simulink model "SecRwLtStHdrstFwdBkwdCtrl"  (R2018b)
settings: Solver=FixedStepDiscrete  StartTime=0.0  StopTime=10.0  FixedStep=0.01  RelTol=1e-3
undefined symbols (not defined in the file or in its folder): KeSMSuMdMotFinshdTm_Val, KeSMSuMdRetryTm1_Val, KeSMSuModeReqDurgTm_Val, KeSMSwSecRwLtStHdrstFwdBkwdEnTrigBitMask_Val
libraries: StCtrlLib x1
settings Model: Creator=sn2xws  LastModifiedBy=sn2xws
settings DataIOCC: SaveFormat=StructureWithTime
settings OptimizationCC: DefaultParameterBehavior=Inlined  EnhancedBackFolding=on  PassReuseOutputArgsAs=Individual arguments  ZeroExternalMemoryAtStartup=off  ZeroInternalMemoryAtStartup=off  OptimizeBlockOrder=speed  DifferentSizesBufferReuse=on  OptimizationCustomize=off
settings DebuggingCC: ParameterTunabilityLossMsg=error
settings ModelReferenceCC: ModelReferenceNumInstancesAllowed=Single
settings SFSimCC: MATLABDynamicMemAlloc=off
settings RTWCC: SystemTargetFile=autosar.tlc  GenCodeOnly=on  TemplateMakefile=ert_default_tmf  Description=AUTOSAR  GenerateReport=on  IncludeHyperlinkInReport=on  LaunchReport=on  GenerateTraceInfo=on  GenerateTraceReport=on  GenerateTraceReportSl=on  GenerateTraceReportSf=on  GenerateTraceReportEml=on
settings CodeAppCC: ForceParamTrailComments=on  IgnoreCustomStorageClasses=off  OperatorAnnotations=on  SimulinkDataObjDesc=on  SFDataObjDesc=on  InsertBlockDesc=on
settings STFCustomTargetCC: TargetLangStandard=C99 (ISO)  MultiwordLength=256  ParMdlRefBuildCompliant=on  CompOptLevelCompliant=on  IncludeMdlTerminateFcn=off  CombineOutputUpdateFcns=on  SuppressErrorStatus=on  ERTCustomFileBanners=on  SupportNonFinite=off  SupportComplex=off  SupportContinuousTime=off  SupportNonInlinedSFcns=off  RemoveResetFunc=on  MATLABClassNameForMDSCustomization=Simulink.SoftwareTarget.ERTCustomization  AutosarCompliant=on  UseToolchainInfoCompliant=on  LookupTableObjectStructAxisOrder=2,1,3,4,...  LUTObjectStructOrderEvenSpacing=Size,Table,Breakpoints  SystemTargetFile=autosar.tlc
settings ERTTargetCC: TargetLangStandard=C99 (ISO)  ConcurrentExecutionCompliant=off  IncludeMdlTerminateFcn=off  SuppressErrorStatus=on  SupportNonFinite=off  SupportComplex=off  ModelStepFunctionPrototypeControlCompliant=off  CPPClassGenCompliant=off  AutosarCompliant=on  LookupTableObjectStructAxisOrder=2,1,3,4,...  LUTObjectStructOrderEvenSpacing=Size,Table,Breakpoints  InlinedParameterPlacement=NonHierarchical  ERTCustomFileTemplate=example_file_process.tlc  ERTFilePackagingFormat=Compact

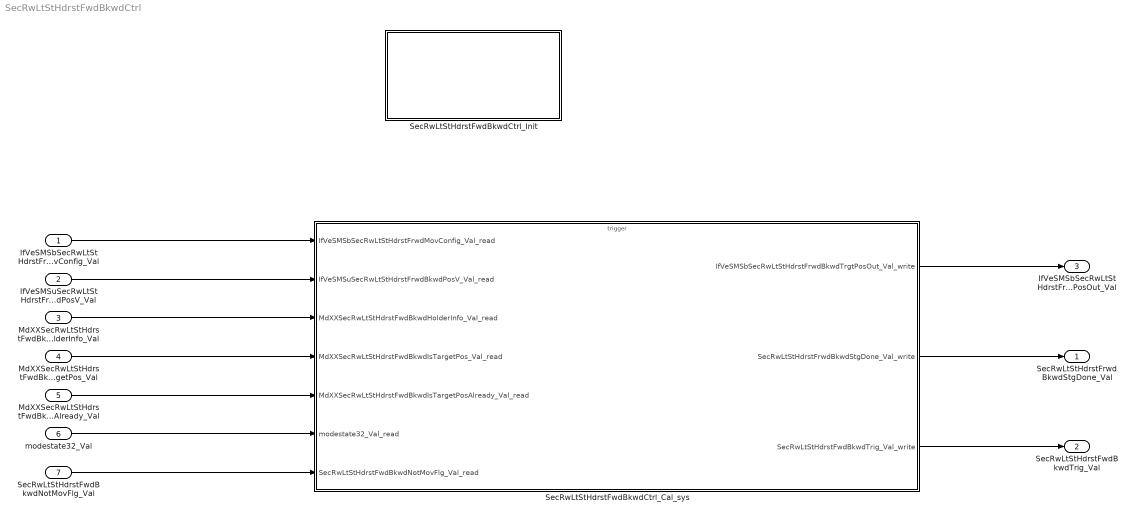
== system SecRwLtStHdrstFwdBkwdCtrl ==
  IfVeSMSbSecRwLtStHdrstFrwdMovConfig_Val : Inport  OutDataTypeStr=boolean  PortDimensions=1
  IfVeSMSuSecRwLtStHdrstFrwdBkwdPosV_Val : Inport  Port=2  OutDataTypeStr=boolean  PortDimensions=1
  MdXXSecRwLtStHdrstFwdBkwdHolderInfo_Val : Inport  Port=3  OutDataTypeStr=uint32  PortDimensions=1
  MdXXSecRwLtStHdrstFwdBkwdIsTargetPos_Val : Inport  Port=4  OutDataTypeStr=uint32  PortDimensions=1
  MdXXSecRwLtStHdrstFwdBkwdIsTargetPosAlready_Val : Inport  Port=5  OutDataTypeStr=uint32  PortDimensions=1
  modestate32_Val : Inport  Port=6  OutDataTypeStr=uint32  PortDimensions=1
  SecRwLtStHdrstFwdBkwdNotMovFlg_Val : Inport  Port=7  OutDataTypeStr=boolean  PortDimensions=1
  SecRwLtStHdrstFwdBkwdCtrl_Cal_sys : Subsystem
  SecRwLtStHdrstFwdBkwdCtrl_Init : Subsystem
  SecRwLtStHdrstFrwdBkwdStgDone_Val : Outport  OutDataTypeStr=boolean  PortDimensions=1
  SecRwLtStHdrstFwdBkwdTrig_Val : Outport  Port=2  OutDataTypeStr=boolean  PortDimensions=1
  IfVeSMSbSecRwLtStHdrstFrwdBkwdTrgtPosOut_Val : Outport  Port=3  OutDataTypeStr=boolean  PortDimensions=1
  wires:
  IfVeSMSbSecRwLtStHdrstFrwdMovConfig_Val/1 -> SecRwLtStHdrstFwdBkwdCtrl_Cal_sys/1(IfVeSMSbSecRwLtStHdrstFrwdMovConfig_Val_read)
  IfVeSMSuSecRwLtStHdrstFrwdBkwdPosV_Val/1 -> SecRwLtStHdrstFwdBkwdCtrl_Cal_sys/2(IfVeSMSuSecRwLtStHdrstFrwdBkwdPosV_Val_read)
  MdXXSecRwLtStHdrstFwdBkwdHolderInfo_Val/1 -> SecRwLtStHdrstFwdBkwdCtrl_Cal_sys/3(MdXXSecRwLtStHdrstFwdBkwdHolderInfo_Val_read)
  MdXXSecRwLtStHdrstFwdBkwdIsTargetPos_Val/1 -> SecRwLtStHdrstFwdBkwdCtrl_Cal_sys/4(MdXXSecRwLtStHdrstFwdBkwdIsTargetPos_Val_read)
  MdXXSecRwLtStHdrstFwdBkwdIsTargetPosAlready_Val/1 -> SecRwLtStHdrstFwdBkwdCtrl_Cal_sys/5(MdXXSecRwLtStHdrstFwdBkwdIsTargetPosAlready_Val_read)
  modestate32_Val/1 -> SecRwLtStHdrstFwdBkwdCtrl_Cal_sys/6(modestate32_Val_read)
  SecRwLtStHdrstFwdBkwdNotMovFlg_Val/1 -> SecRwLtStHdrstFwdBkwdCtrl_Cal_sys/7(SecRwLtStHdrstFwdBkwdNotMovFlg_Val_read)
  SecRwLtStHdrstFwdBkwdCtrl_Cal_sys/1(IfVeSMSbSecRwLtStHdrstFrwdBkwdTrgtPosOut_Val_write) -> IfVeSMSbSecRwLtStHdrstFrwdBkwdTrgtPosOut_Val/1
  SecRwLtStHdrstFwdBkwdCtrl_Cal_sys/2(SecRwLtStHdrstFrwdBkwdStgDone_Val_write) -> SecRwLtStHdrstFrwdBkwdStgDone_Val/1
  SecRwLtStHdrstFwdBkwdCtrl_Cal_sys/3(SecRwLtStHdrstFwdBkwdTrig_Val_write) -> SecRwLtStHdrstFwdBkwdTrig_Val/1

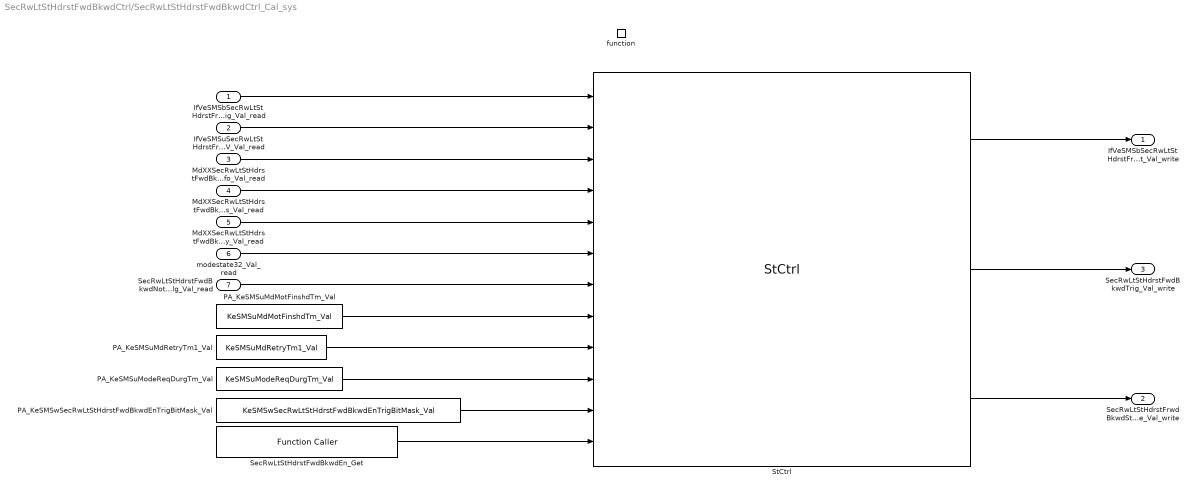
== system SecRwLtStHdrstFwdBkwdCtrl/SecRwLtStHdrstFwdBkwdCtrl_Cal_sys ==
  IfVeSMSbSecRwLtStHdrstFrwdMovConfig_Val_read : Inport
  IfVeSMSuSecRwLtStHdrstFrwdBkwdPosV_Val_read : Inport  Port=2
  MdXXSecRwLtStHdrstFwdBkwdHolderInfo_Val_read : Inport  Port=3
  MdXXSecRwLtStHdrstFwdBkwdIsTargetPos_Val_read : Inport  Port=4
  MdXXSecRwLtStHdrstFwdBkwdIsTargetPosAlready_Val_read : Inport  Port=5
  modestate32_Val_read : Inport  Port=6
  SecRwLtStHdrstFwdBkwdNotMovFlg_Val_read : Inport  Port=7
  function : TriggerPort  TriggerType=function-call  IsSimulinkFunction=on  FunctionName=SecRwLtStHdrstFwdBkwdCtrl_Cal  VariantControl=(inherit)
  PA_KeSMSuMdMotFinshdTm_Val : Constant  Value=KeSMSuMdMotFinshdTm_Val
  PA_KeSMSuMdRetryTm1_Val : Constant  Value=KeSMSuMdRetryTm1_Val
  PA_KeSMSuModeReqDurgTm_Val : Constant  Value=KeSMSuModeReqDurgTm_Val
  PA_KeSMSwSecRwLtStHdrstFwdBkwdEnTrigBitMask_Val : Constant  Value=KeSMSwSecRwLtStHdrstFwdBkwdEnTrigBitMask_Val
  SecRwLtStHdrstFwdBkwdEn_Get : FunctionCaller  FunctionPrototype=data = SecRwLtStHdrstFwdBkwdEn_Get()  OutputArgumentSpecifications=uint32(1)
  StCtrl : StCtrlLib/StCtrl  SystemSampleTime=-1
  IfVeSMSbSecRwLtStHdrstFrwdBkwdTrgtPosOut_Val_write : Outport
      settings: EnsureOutportIsVirtual=on
  SecRwLtStHdrstFrwdBkwdStgDone_Val_write : Outport  Port=2
      settings: EnsureOutportIsVirtual=on
  SecRwLtStHdrstFwdBkwdTrig_Val_write : Outport  Port=3
      settings: EnsureOutportIsVirtual=on
  wires:
  StCtrl/2 -> SecRwLtStHdrstFwdBkwdTrig_Val_write/1
  StCtrl/1 -> IfVeSMSbSecRwLtStHdrstFrwdBkwdTrgtPosOut_Val_write/1
  StCtrl/3 -> SecRwLtStHdrstFrwdBkwdStgDone_Val_write/1
  PA_KeSMSwSecRwLtStHdrstFwdBkwdEnTrigBitMask_Val/1 -> StCtrl/11
  SecRwLtStHdrstFwdBkwdEn_Get/1 -> StCtrl/12
  PA_KeSMSuMdMotFinshdTm_Val/1 -> StCtrl/8
  PA_KeSMSuModeReqDurgTm_Val/1 -> StCtrl/10
  PA_KeSMSuMdRetryTm1_Val/1 -> StCtrl/9
  IfVeSMSbSecRwLtStHdrstFrwdMovConfig_Val_read/1 -> StCtrl/1
  IfVeSMSuSecRwLtStHdrstFrwdBkwdPosV_Val_read/1 -> StCtrl/2
  MdXXSecRwLtStHdrstFwdBkwdHolderInfo_Val_read/1 -> StCtrl/3
  MdXXSecRwLtStHdrstFwdBkwdIsTargetPos_Val_read/1 -> StCtrl/4
  MdXXSecRwLtStHdrstFwdBkwdIsTargetPosAlready_Val_read/1 -> StCtrl/5
  modestate32_Val_read/1 -> StCtrl/6
  SecRwLtStHdrstFwdBkwdNotMovFlg_Val_read/1 -> StCtrl/7

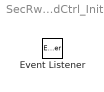
== system SecRwLtStHdrstFwdBkwdCtrl/SecRwLtStHdrstFwdBkwdCtrl_Init ==
  Event Listener : EventListener  EventName=reset
